simulink model "IEEE24bus_simplified"  (R2019b)
settings: Solver=ode23tb  StartTime=0.0  StopTime=100  MaxStep=1/60  RelTol=1e-4  AbsTol=1e-3  EnableMultiTasking=on
PreLoadFcn:
  | RTS96_data
values from neighbouring files (symbols this model uses):
  Efmax = 5    [IEEE24_bus.m]    (also in IEEE24bus_simplified_benchmark.m)
  Efmin = -5    [IEEE24_bus.m]    (also in IEEE24bus_simplified_benchmark.m)
  EXc_sys = [     0.06  25  0.2    0.0505  0.5685   0 0   0.091  0.35 ... (first row only)    [IEEE24bus_simplified_benchmark.m]
  FH1 = 12    [IEEE24bus_simplified_benchmark.m]
  FI1 = .9    (= 0.9)    [IEEE24bus_simplified_benchmark.m]
  FL1 = .1    (= 0.1)    [IEEE24bus_simplified_benchmark.m]
  KH1 = 100    [IEEE24bus_simplified_benchmark.m]
  KI1 = 1    [IEEE24_bus.m]    (also in IEEE24bus_simplified_benchmark.m = 20)
  KL1 = 10    [IEEE24bus_simplified_benchmark.m]
undefined symbols (not defined in the file or in its folder): D1, Delta
libraries: powerlib x157, sps_avr x11, powerlib_extras x1
(part 2 of 3)

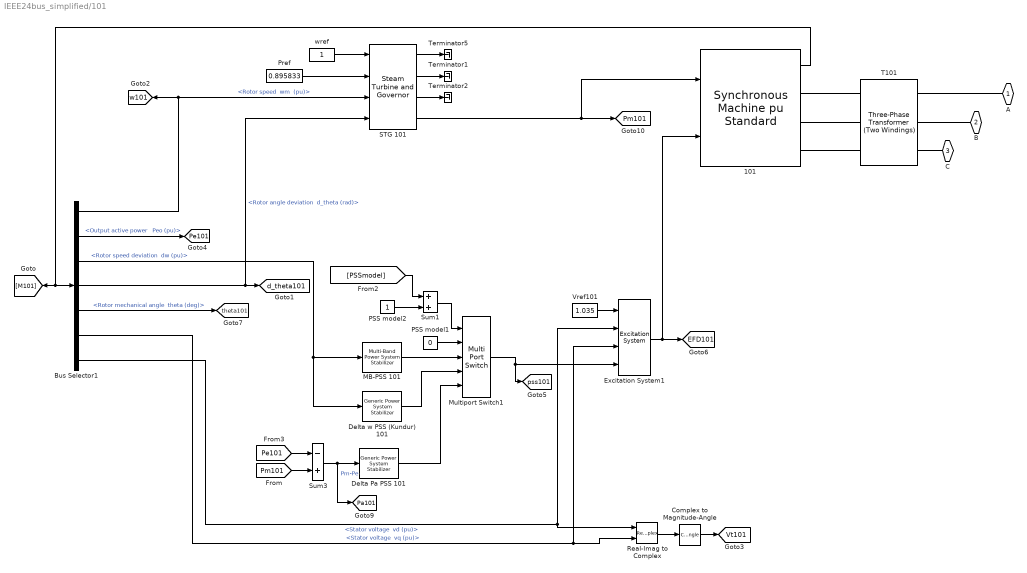
== system IEEE24bus_simplified/101 ==
  101 : powerlib/Machines/Synchronous Machine pu Standard  RequirementInfo={'other' '..\..\..\..\public\documents\just test.xlsx' '@Simulink_requirement_item_1' 'true' '' '' } %GIDa_22814801_0845_46e3_8641_b30c20268729  PresetModel=No  MechanicalLoad=Mechanical power Pm  ShowDetailedParameters=on  RotorType=Round  Units=per unit standard parameters  MeasurementBus=off  NominalParameters="[ 192E6  18000  60]"  Reactances1="[ 1.65  0.232  0.171  1.59  0.38  0.171  0.102 ]"  Reactances2="[ 1.651, 0.232, 0.171, 1.590,  0.171,  0.102 ]"  dAxisTimeConstants=Open-circuit  qAxisTimeConstants=Open-circuit  TimeConstants1="[  5.9  0.033  0.023  ]"  TimeConstants2="[ 5.9  0.033  0.735  0.078 ]"  TimeConstants3="[  5.9  0.033  0.023  ]"  TimeConstants4=[ 8.0, 0.03, 0.3371, 0.0295 ]  TimeConstants5=[ 1.01, 0.053, 0.1 ]  TimeConstants6=[ 1.3201, 0.023, 1.0, 0.07 ]  TimeConstants7="[  1.01  0.053  0.051266  ]"  TimeConstants8=[ 1.3201, 0.0231, 0.3371, 0.0295 ]  StatorResistance=0.0026  Mechanical="[ 960/233 0  4 ]"  PolePairs=4  InitialConditions=[0 -54.7243 0.868552 0.868552 0.868552 -19.5576 -139.558 100.442 1.8373]  SetSaturation=off  Saturation=[0.6404,0.7127,0.8441,0.9214,0.9956,1.082,1.19,1.316,1.457;0.7,0.7698,0.8872,0.9466,0.9969,1.046,1.1,1.151,1.201]  LoadFlowParameters=[1 172000000 18630 0 0]  TsPowergui=0  TsBlock=-1  IterativeModel=Forward Euler  IterativeDiscreteModel=Trapezoidal non iterative  BusType=PV  Pref=172E6  Qref=0  Qmin=-50E6  Qmax=80e6  PLF=0  QLF=0
      settings: SourceProductName=Simscape Electrical
  Bus Selector1 : BusSelector  OutputSignals="Mechanical.Rotor speed  wm  (pu),Output active power   Peo (pu),Mechanical.Rotor speed deviation  dw (pu),Mechanical.Rotor angle deviation  d_theta (rad),Mechanical.Rotor mechanical angle  theta (deg),dq0 components.Stator voltage  vq (pu),dq0 components.Stator voltage  vd (pu)"
  Complex to Magnitude-Angle : ComplexToMagnitudeAngle  Output=Magnitude
  Delta Pa PSS 101 : powerlib/Machines/Generic Power System Stabilizer  Tsensor=15e-3  K=2.5*1.25  Twashout=1  Tleadlag1=[60e-3 1]  Tleadlag2=[0 0]  VSlimits=[-0.15 0.15]  Vinit=0  Plot_On=off  MagdB_On=on  FreqRange=logspace(-2,2,500)
      settings: SourceProductName=Simscape Electrical  SourceProductBaseCode=PS
  Delta w PSS (Kundur) 101 : powerlib/Machines/Generic Power System Stabilizer  Tsensor=15e-3  K=30  Twashout=10  Tleadlag1=[50e-3 20e-3]  Tleadlag2=[3 5.4]  VSlimits=[-0.15 0.15]  Vinit=0  Plot_On=off  MagdB_On=on  FreqRange=logspace(-2,2,500)
      settings: SourceProductName=Simscape Electrical  SourceProductBaseCode=PS
  Excitation System1 : sps_avr/Excitation System  tr=EXc_sys(1,1)  reg="[ EXc_sys(1,2)   EXc_sys(1,3) ]"  exc="[ EXc_sys(1,4)  EXc_sys(1,5)]"  tgr="[ EXc_sys(1,6)  EXc_sys(1,7) ]"  damp="[ EXc_sys(1,8)   EXc_sys(1,9)]"  sat=[ 0, 0 ]  lim="[ Efmin Efmax   0 ]"  v0=[1.035,1.8373]
      settings: SourceProductName=Simscape Electrical  SourceProductBaseCode=PS
  "MB-PSS 101 " : powerlib/Machines/Multi-Band Power System Stabilizer  OperationMode=Simplified settings  Kg=G1  GL=[FL1 KL1]  GI=[FI1 KI1]  GH=[FH1 KH1]  GLd=[66 66 9.4]  TcLF=[1.667 2 0 0 0 0 2 2.4 0 0 0 0 1 1]  GId=[66 66 47.6]  TcIF=[1 1 0.25 0.3 0 0 1 1 0.3 0.36 0 0 0 0]  GHd=[66 66 233]  TcHF="[0.01 0.012 0 0 0 0  0.012 0.0144 0 0 0 0 1 1]"  LIM=[.075 .15 .15 .15]  Plot_On=off  MagdB_On=off  FreqRange=logspace(-2,2,500)
      settings: SourceProductName=Simscape Electrical  SourceProductBaseCode=PS
  Multiport Switch1 : MultiPortSwitch  Inputs=4  InputSameDT=on
  PSS model1 : Constant  Value=0
  PSS model2 : Constant
  Pref : Constant  Value=0.895833
  Real-Imag to Complex : RealImagToComplex
  STG 101 : powerlib/Machines/Steam Turbine and Governor  gentype=Tandem-compound (single mass)  reg1="[ 1  0.05    0 ]"  reg2="[ 0.001  0.15 ]"  reg3="[ -0.1  0.1  0  4.496 ]"  N=3600  turb1="[ 0  10   3.3   0.5   ]"  turb2="[   0   0.36    0.36   0.28   ]"  HA="[ 0.046  1.430  1.465   0.192 ]"  KA="[ 90.44  53.88  64.59   62.94  ]"  DA="[ 0.0115  0.3575  0.3663   0.0137  ]"  ini1=0.897795  ini2=[0.779316,-31.4247]
      settings: SourceProductName=Simscape Electrical  SourceProductBaseCode=PS
  Sum1 : Sum  SaturateOnIntegerOverflow=on  InputSameDT=on  OutDataTypeStr=Inherit: Same as first input
  Sum3 : Sum  Inputs=-+  SaturateOnIntegerOverflow=on  InputSameDT=on  OutDataTypeStr=Inherit: Same as first input
  T101 : powerlib/Elements/Three-Phase Transformer (Two Windings)  Winding1Connection=Yg  Winding2Connection=Delta (D1)  CoreType=Three single-phase transformers  SetSaturation=off  Hysteresis=off  DataFile='hysteresis'  SetInitialFlux=off  Measurements=None  UNITS=pu  NominalPower=[ 236E6 , 60 ]  Winding1=[ 138e3 , 0, 0.13 ]  Winding2=[ 18e3 , 1e-6, 0 ]  Rm=500  Lm=500  L0=0.5  Saturation=[ 0,0 ; 0.0024,1.2 ; 1.0,1.52 ]  InitialFluxes=[ 0.8 , -0.8 , 0.7 ]  BreakLoop=off  DiscreteSolver=Trapezoidal iterative  DataType=off  TransfoNumber=0
      settings: SourceProductName=Simscape Electrical
  Terminator1 : Terminator
  Terminator2 : Terminator
  Terminator5 : Terminator
  Vref101 : Constant  Value=1.035
  wref : Constant
  A : PMIOPort  Side=Left
  B : PMIOPort  Port=2  Side=Left
  C : PMIOPort  Port=3  Side=Left
  tag scope: EFD101=global, Pa101=global, Pe101=global, Pm101=global, Vt101=global, d_theta101=global, pss101=global, theta101=global, w101=global
  wires:
  Bus Selector1/6 -> Real-Imag to Complex/2, Excitation System1/3  "<Stator voltage  vq (pu)>"
  Bus Selector1/7 -> Real-Imag to Complex/1, Excitation System1/2  "<Stator voltage  vd (pu)>"
  wref/1 -> STG 101/1
  Vref101/1 -> Excitation System1/1
  Pref/1 -> STG 101/2
  Bus Selector1/4 -> STG 101/4, [d_theta101]  "<Rotor angle deviation  d_theta (rad)>"
  101/1 -> Bus Selector1/1, [M101]
  STG 101/1 -> Terminator5/1
  Bus Selector1/1 -> STG 101/3, [w101]  "<Rotor speed  wm  (pu)>"
  Real-Imag to Complex/1 -> Complex to Magnitude-Angle/1
  Complex to Magnitude-Angle/1 -> [Vt101]
  PSS model2/1 -> Sum1/2
  Sum1/1 -> Multiport Switch1/1
  Excitation System1/1 -> 101/2, [EFD101]
  Multiport Switch1/1 -> Excitation System1/4, [pss101]
  [PSSmodel] -> Sum1/1
  PSS model1/1 -> Multiport Switch1/2
  "MB-PSS 101 "/1 -> Multiport Switch1/3
  Bus Selector1/5 -> [theta101]  "<Rotor mechanical angle  theta (deg)>"
  Bus Selector1/2 -> [Pe101]  "<Output active power   Peo (pu)>"
  STG 101/2 -> Terminator1/1
  STG 101/3 -> Terminator2/1
  Bus Selector1/3 -> Delta w PSS (Kundur) 101/1, "MB-PSS 101 "/1  "<Rotor speed deviation  dw (pu)>"
  Sum3/1 -> [Pa101], Delta Pa PSS 101/1  "Pm-Pe"
  Delta Pa PSS 101/1 -> Multiport Switch1/5
  Delta w PSS (Kundur) 101/1 -> Multiport Switch1/4
  [Pm101] -> Sum3/2
  [Pe101] -> Sum3/1
  STG 101/4 -> 101/1, [Pm101]
  connections:
  101/RConn2 -- T101/RConn2
  101/RConn1 -- T101/RConn1
  101/RConn3 -- T101/RConn3
  C/RConn1 -- T101/LConn3
  B/RConn1 -- T101/LConn2
  A/RConn1 -- T101/LConn1

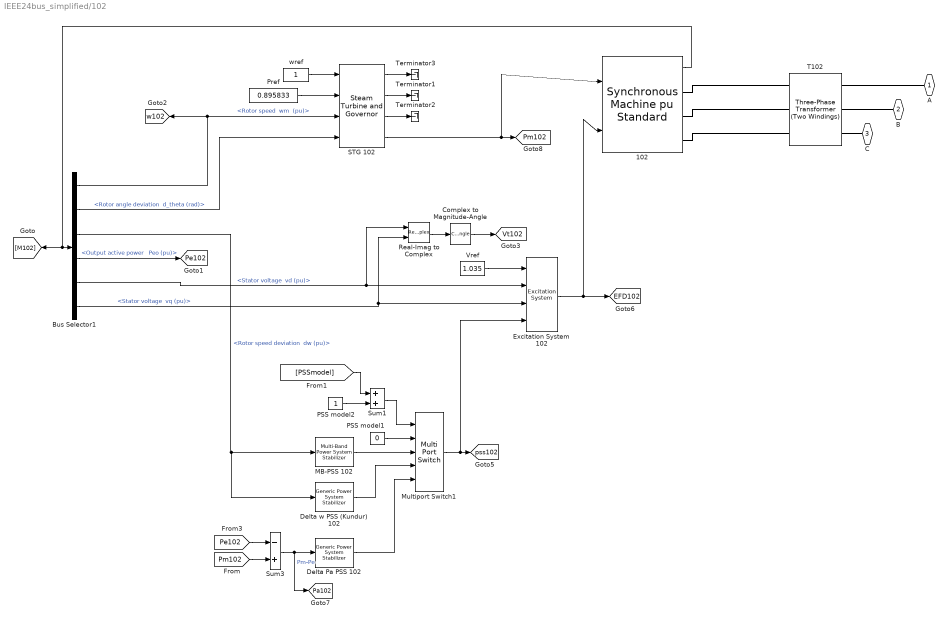
== system IEEE24bus_simplified/102 ==
  102 : powerlib/Machines/Synchronous Machine pu Standard  PresetModel=No  MechanicalLoad=Mechanical power Pm  ShowDetailedParameters=on  RotorType=Round  Units=per unit standard parameters  MeasurementBus=off  NominalParameters="[ 192E6  18000  60]"  Reactances1="[ 1.65  0.232  0.171  1.59  0.38  0.171  0.102 ]"  Reactances2="[ 1.651, 0.232, 0.171, 1.590,  0.171,  0.102 ]"  dAxisTimeConstants=Open-circuit  qAxisTimeConstants=Open-circuit  TimeConstants1="[  5.9  0.033  0.023  ]"  TimeConstants2="[ 5.9  0.033  0.735  0.078 ]"  TimeConstants3="[  5.9  0.033  0.023  ]"  TimeConstants4=[ 8.0, 0.03, 0.3371, 0.0295 ]  TimeConstants5=[ 1.01, 0.053, 0.1 ]  TimeConstants6=[ 1.3201, 0.023, 1.0, 0.07 ]  TimeConstants7="[  1.01  0.053  0.051266  ]"  TimeConstants8=[ 1.3201, 0.0231, 0.3371, 0.0295 ]  StatorResistance=0.0026  Mechanical="[ 960/233 0  4 ]"  PolePairs=4  InitialConditions=[0 -53.6767 0.866594 0.866594 0.866594 -17.7339 -137.734 102.266 1.80706]  SetSaturation=off  Saturation=[0.6404,0.7127,0.8441,0.9214,0.9956,1.082,1.19,1.316,1.457;0.7,0.7698,0.8872,0.9466,0.9969,1.046,1.1,1.151,1.201]  LoadFlowParameters=[1 172000000 18630 0 0]  TsPowergui=0  TsBlock=-1  IterativeModel=Forward Euler  IterativeDiscreteModel=Trapezoidal non iterative  BusType=PV  Pref=172E6  Qref=0  Qmin=-50e6  Qmax=80E6  PLF=0  QLF=0
      settings: SourceProductName=Simscape Electrical
  Bus Selector1 : BusSelector  OutputSignals="Mechanical.Rotor speed  wm  (pu),Mechanical.Rotor angle deviation  d_theta (rad),Mechanical.Rotor speed deviation  dw (pu),Output active power   Peo (pu),dq0 components.Stator voltage  vd (pu),dq0 components.Stator voltage  vq (pu)"
  Complex to Magnitude-Angle : ComplexToMagnitudeAngle  Output=Magnitude
  Delta Pa PSS 102 : powerlib/Machines/Generic Power System Stabilizer  Tsensor=15e-3  K=2.5*1.25  Twashout=1  Tleadlag1=[60e-3 1]  Tleadlag2=[0 0]  VSlimits=[-0.15 0.15]  Vinit=0  Plot_On=off  MagdB_On=on  FreqRange=logspace(-2,2,500)
      settings: SourceProductName=Simscape Electrical  SourceProductBaseCode=PS
  Delta w PSS (Kundur) 102 : powerlib/Machines/Generic Power System Stabilizer  Tsensor=15e-3  K=30  Twashout=10  Tleadlag1=[50e-3 20e-3]  Tleadlag2=[3 5.4]  VSlimits=[-0.15 0.15]  Vinit=0  Plot_On=off  MagdB_On=on  FreqRange=logspace(-2,2,500)
      settings: SourceProductName=Simscape Electrical  SourceProductBaseCode=PS
  Excitation System 102 : sps_avr/Excitation System  tr=EXc_sys(2,1)  reg="[ EXc_sys(2,2)   EXc_sys(2,3) ]"  exc="[ EXc_sys(2,4)  EXc_sys(2,5)]"  tgr="[ EXc_sys(2,6)  EXc_sys(2,7) ]"  damp="[ EXc_sys(2,8)   EXc_sys(2,9)]"  sat=[ 0, 0 ]  lim="[ Efmin Efmax   0 ]"  v0=[1.035,1.80706]
      settings: SourceProductName=Simscape Electrical  SourceProductBaseCode=PS
  "MB-PSS 102 " : powerlib/Machines/Multi-Band Power System Stabilizer  OperationMode=Simplified settings  Kg=G1  GL=[FL1 KL1]  GI=[FI1 KI1]  GH=[FH1 KH1]  GLd=[66 66 9.4]  TcLF=[1.667 2 0 0 0 0 2 2.4 0 0 0 0 1 1]  GId=[66 66 47.6]  TcIF=[1 1 0.25 0.3 0 0 1 1 0.3 0.36 0 0 0 0]  GHd=[66 66 233]  TcHF="[0.01 0.012 0 0 0 0  0.012 0.0144 0 0 0 0 1 1]"  LIM=[.075 .15 .15 .15]  Plot_On=off  MagdB_On=off  FreqRange=logspace(-2,2,500)
      settings: SourceProductName=Simscape Electrical  SourceProductBaseCode=PS
  Multiport Switch1 : MultiPortSwitch  Inputs=4  InputSameDT=on
  PSS model1 : Constant  Value=0
  PSS model2 : Constant
  Pref : Constant  Value=0.895833
  Real-Imag to Complex : RealImagToComplex
  STG 102 : powerlib/Machines/Steam Turbine and Governor  gentype=Tandem-compound (single mass)  reg1="[ 1  0.05    0 ]"  reg2="[ 0.001  0.15 ]"  reg3="[ -0.1  0.1  0  4.496 ]"  N=3600  turb1="[ 0  10   3.3   0.5   ]"  turb2="[   0   0.36    0.36   0.28   ]"  HA="[ 0.046  1.430  1.465   0.192 ]"  KA="[ 90.44  53.88  64.59   62.94  ]"  DA="[ 0.0115  0.3575  0.3663   0.0137  ]"  ini1=0.897786  ini2=[0.779316,-31.4247]
      settings: SourceProductName=Simscape Electrical  SourceProductBaseCode=PS
  Sum1 : Sum  SaturateOnIntegerOverflow=on  InputSameDT=on  OutDataTypeStr=Inherit: Same as first input
  Sum3 : Sum  Inputs=-+  SaturateOnIntegerOverflow=on  InputSameDT=on  OutDataTypeStr=Inherit: Same as first input
  T102 : powerlib/Elements/Three-Phase Transformer (Two Windings)  Winding1Connection=Yg  Winding2Connection=Delta (D1)  CoreType=Three single-phase transformers  SetSaturation=off  Hysteresis=off  DataFile='hysteresis'  SetInitialFlux=off  Measurements=None  UNITS=pu  NominalPower="[ 236E6  , 60 ]"  Winding1=[ 138e3 , 0, .13 ]  Winding2=[ 18e3 , 1e-6 , 0 ]  Rm=500  Lm=500  L0=0.5  Saturation=[ 0,0 ; 0.0024,1.2 ; 1.0,1.52 ]  InitialFluxes=[ 0.8 , -0.8 , 0.7 ]  BreakLoop=off  DiscreteSolver=Trapezoidal iterative  DataType=off  TransfoNumber=0
      settings: SourceProductName=Simscape Electrical
  Terminator1 : Terminator
  Terminator2 : Terminator
  Terminator3 : Terminator
  Vref : Constant  Value=1.035
  wref : Constant
  A : PMIOPort  Side=Left
  B : PMIOPort  Port=2  Side=Left
  C : PMIOPort  Port=3  Side=Left
  tag scope: EFD102=global, Pa102=global, Pe102=global, Pm102=global, Vt102=global, pss102=global, w102=global
  wires:
  STG 102/1 -> Terminator3/1
  STG 102/2 -> Terminator1/1
  STG 102/3 -> Terminator2/1
  STG 102/4 -> [Pm102], 102/1
  wref/1 -> STG 102/1
  Pref/1 -> STG 102/2
  102/1 -> [M102], Bus Selector1/1
  Bus Selector1/1 -> [w102], STG 102/3  "<Rotor speed  wm  (pu)>"
  Bus Selector1/2 -> STG 102/4  "<Rotor angle deviation  d_theta (rad)>"
  Vref/1 -> Excitation System 102/1
  Bus Selector1/5 -> Real-Imag to Complex/1, Excitation System 102/2  "<Stator voltage  vd (pu)>"
  Bus Selector1/6 -> Real-Imag to Complex/2, Excitation System 102/3  "<Stator voltage  vq (pu)>"
  PSS model2/1 -> Sum1/2
  Sum1/1 -> Multiport Switch1/1
  Multiport Switch1/1 -> Excitation System 102/4, [pss102]
  [PSSmodel] -> Sum1/1
  PSS model1/1 -> Multiport Switch1/2
  "MB-PSS 102 "/1 -> Multiport Switch1/3
  Bus Selector1/4 -> [Pe102]  "<Output active power   Peo (pu)>"
  Excitation System 102/1 -> 102/2, [EFD102]
  Real-Imag to Complex/1 -> Complex to Magnitude-Angle/1
  Complex to Magnitude-Angle/1 -> [Vt102]
  Bus Selector1/3 -> Delta w PSS (Kundur) 102/1, "MB-PSS 102 "/1  "<Rotor speed deviation  dw (pu)>"
  Sum3/1 -> [Pa102], Delta Pa PSS 102/1  "Pm-Pe"
  Delta Pa PSS 102/1 -> Multiport Switch1/5
  Delta w PSS (Kundur) 102/1 -> Multiport Switch1/4
  [Pm102] -> Sum3/2
  [Pe102] -> Sum3/1
  connections:
  102/RConn3 -- T102/RConn3
  102/RConn2 -- T102/RConn2
  102/RConn1 -- T102/RConn1
  A/RConn1 -- T102/LConn1
  C/RConn1 -- T102/LConn3
  B/RConn1 -- T102/LConn2

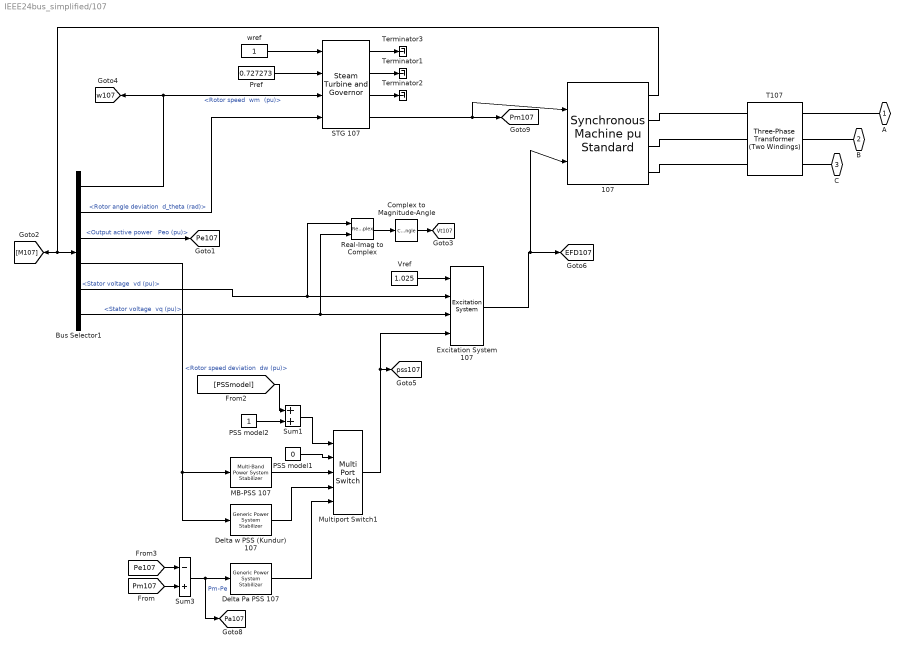
== system IEEE24bus_simplified/107 ==
  107 : powerlib/Machines/Synchronous Machine pu Standard  PresetModel=No  MechanicalLoad=Mechanical power Pm  ShowDetailedParameters=on  RotorType=Round  Units=per unit standard parameters  MeasurementBus=off  NominalParameters="[ 330E6  20000   60]"  Reactances1="[ 1.95  0.317  .2  1.92  1.12  .2  0.199 ]"  Reactances2="[ 1.9, 0.317, 0.001, 1.9,  0.001,  0.199 ]"  dAxisTimeConstants=Open-circuit  qAxisTimeConstants=Open-circuit  TimeConstants1="[  6  0.01  0.01  ]"  TimeConstants2="[ 6 .04  1.5  .08 ]"  TimeConstants3="[  6  0.01  0.01  ]"  TimeConstants4=[ 8.0, 0.03, 0.3371, 0.0295 ]  TimeConstants5=[ 1.01, 0.053, 0.1 ]  TimeConstants6=[ 1.3201, 0.023, 1.0, 0.07 ]  TimeConstants7="[  1.01  0.053  0.051266  ]"  TimeConstants8=[ 1.3201, 0.0231, 0.3371, 0.0295 ]  StatorResistance=0.0015  Mechanical="[ 992/330  0  4 ]"  PolePairs=4  InitialConditions=[0 -63.9537 0.747482 0.747482 0.747482 -34.958 -154.958 85.042 2.02909]  SetSaturation=off  Saturation=[0.6404,0.7127,0.8441,0.9214,0.9956,1.082,1.19,1.316,1.457;0.7,0.7698,0.8872,0.9466,0.9969,1.046,1.1,1.151,1.201]  LoadFlowParameters=[1 240000000 20500 0 0]  TsPowergui=0  TsBlock=-1  IterativeModel=Forward Euler  IterativeDiscreteModel=Trapezoidal non iterative  BusType=PV  Pref=240E6  Qref=0  Qmin=0  Qmax=180E6  PLF=0  QLF=0
      settings: SourceProductName=Simscape Electrical
  Bus Selector1 : BusSelector  OutputSignals="Mechanical.Rotor speed  wm  (pu),Mechanical.Rotor angle deviation  d_theta (rad),Output active power   Peo (pu),Mechanical.Rotor speed deviation  dw (pu),dq0 components.Stator voltage  vd (pu),dq0 components.Stator voltage  vq (pu)"
  Complex to Magnitude-Angle : ComplexToMagnitudeAngle  Output=Magnitude
  Delta Pa PSS 107 : powerlib/Machines/Generic Power System Stabilizer  Tsensor=15e-3  K=2.5*1.25  Twashout=1  Tleadlag1=[60e-3 1]  Tleadlag2=[0 0]  VSlimits=[-0.15 0.15]  Vinit=0  Plot_On=off  MagdB_On=on  FreqRange=logspace(-2,2,500)
      settings: SourceProductName=Simscape Electrical  SourceProductBaseCode=PS
  Delta w PSS (Kundur) 107 : powerlib/Machines/Generic Power System Stabilizer  Tsensor=15e-3  K=30  Twashout=10  Tleadlag1=[50e-3 20e-3]  Tleadlag2=[3 5.4]  VSlimits=[-0.15 0.15]  Vinit=0  Plot_On=off  MagdB_On=on  FreqRange=logspace(-2,2,500)
      settings: SourceProductName=Simscape Electrical  SourceProductBaseCode=PS
  Excitation System 107 : sps_avr/Excitation System  tr=EXc_sys(3,1)  reg="[ EXc_sys(3,2)   EXc_sys(3,3) ]"  exc="[ EXc_sys(3,4)  EXc_sys(3,5)]"  tgr="[ EXc_sys(3,6)  EXc_sys(3,7) ]"  damp="[ EXc_sys(3,8)   EXc_sys(3,9)]"  sat=[ 0, 0 ]  lim="[ Efmin Efmax   0 ]"  v0=[1.025,2.02909]
      settings: SourceProductName=Simscape Electrical  SourceProductBaseCode=PS
  MB-PSS 107 : powerlib/Machines/Multi-Band Power System Stabilizer  OperationMode=Simplified settings  Kg=G1  GL=[FL1 KL1]  GI=[FI1 KI1]  GH=[FH1 KH1]  GLd=[66 66 9.4]  TcLF=[1.667 2 0 0 0 0 2 2.4 0 0 0 0 1 1]  GId=[66 66 47.6]  TcIF=[1 1 0.25 0.3 0 0 1 1 0.3 0.36 0 0 0 0]  GHd=[66 66 233]  TcHF="[0.01 0.012 0 0 0 0  0.012 0.0144 0 0 0 0 1 1]"  LIM=[.075 .15 .15 .15]  Plot_On=off  MagdB_On=off  FreqRange=logspace(-2,2,500)
      settings: SourceProductName=Simscape Electrical  SourceProductBaseCode=PS
  Multiport Switch1 : MultiPortSwitch  Inputs=4  InputSameDT=on
  PSS model1 : Constant  Value=0
  PSS model2 : Constant
  Pref : Constant  Value=0.727273
  Real-Imag to Complex : RealImagToComplex
  STG 107 : powerlib/Machines/Steam Turbine and Governor  gentype=Tandem-compound (single mass)  reg1="[ 1  0.05    0 ]"  reg2="[ 0.001  0.15 ]"  reg3="[ -0.1  0.1  0  4.496 ]"  N=3600  turb1="[ 0  10   3.3   0.5   ]"  turb2="[   0   0.36    0.36   0.28   ]"  HA="[ 0.046  1.430  1.465   0.192 ]"  KA="[ 90.44  53.88  64.59   62.94  ]"  DA="[ 0.0115  0.3575  0.3663   0.0137  ]"  ini1=0.728111  ini2=[0.779316,-31.4247]
      settings: SourceProductName=Simscape Electrical  SourceProductBaseCode=PS
  Sum1 : Sum  SaturateOnIntegerOverflow=on  InputSameDT=on  OutDataTypeStr=Inherit: Same as first input
  Sum3 : Sum  Inputs=-+  SaturateOnIntegerOverflow=on  InputSameDT=on  OutDataTypeStr=Inherit: Same as first input
  T107 : powerlib/Elements/Three-Phase Transformer (Two Windings)  Winding1Connection=Yg  Winding2Connection=Delta (D1)  CoreType=Three single-phase transformers  SetSaturation=off  Hysteresis=off  DataFile='hysteresis'  SetInitialFlux=off  Measurements=None  UNITS=pu  NominalPower=[ 354E6 , 60 ]  Winding1="[ 138e3 , 0,  0.13 ]"  Winding2=[ 20e3 , 1e-6 , 0 ]  Rm=500  Lm=500  L0=0.5  Saturation=[ 0,0 ; 0.0024,1.2 ; 1.0,1.52 ]  InitialFluxes=[ 0.8 , -0.8 , 0.7 ]  BreakLoop=off  DiscreteSolver=Trapezoidal iterative  DataType=off  TransfoNumber=0
      settings: SourceProductName=Simscape Electrical
  Terminator1 : Terminator
  Terminator2 : Terminator
  Terminator3 : Terminator
  Vref : Constant  Value=1.025
  wref : Constant
  A : PMIOPort  Side=Left
  B : PMIOPort  Port=2  Side=Left
  C : PMIOPort  Port=3  Side=Left
  tag scope: EFD107=global, Pa107=global, Pe107=global, Pm107=global, Vt107=global, pss107=global, w107=global
  wires:
  Excitation System 107/1 -> 107/2, [EFD107]
  Vref/1 -> Excitation System 107/1
  107/1 -> [M107], Bus Selector1/1
  STG 107/1 -> Terminator3/1
  STG 107/2 -> Terminator1/1
  STG 107/3 -> Terminator2/1
  STG 107/4 -> [Pm107], 107/1
  Pref/1 -> STG 107/2
  wref/1 -> STG 107/1
  Bus Selector1/1 -> [w107], STG 107/3  "<Rotor speed  wm  (pu)>"
  Bus Selector1/2 -> STG 107/4  "<Rotor angle deviation  d_theta (rad)>"
  PSS model2/1 -> Sum1/2
  Sum1/1 -> Multiport Switch1/1
  Multiport Switch1/1 -> Excitation System 107/4, [pss107]
  [PSSmodel] -> Sum1/1
  PSS model1/1 -> Multiport Switch1/2
  MB-PSS 107/1 -> Multiport Switch1/3
  Bus Selector1/3 -> [Pe107]  "<Output active power   Peo (pu)>"
  Bus Selector1/5 -> Real-Imag to Complex/1, Excitation System 107/2  "<Stator voltage  vd (pu)>"
  Bus Selector1/6 -> Real-Imag to Complex/2, Excitation System 107/3  "<Stator voltage  vq (pu)>"
  Real-Imag to Complex/1 -> Complex to Magnitude-Angle/1
  Complex to Magnitude-Angle/1 -> [Vt107]
  Bus Selector1/4 -> Delta w PSS (Kundur) 107/1, MB-PSS 107/1  "<Rotor speed deviation  dw (pu)>"
  Sum3/1 -> [Pa107], Delta Pa PSS 107/1  "Pm-Pe"
  Delta Pa PSS 107/1 -> Multiport Switch1/5
  Delta w PSS (Kundur) 107/1 -> Multiport Switch1/4
  [Pm107] -> Sum3/2
  [Pe107] -> Sum3/1
  connections:
  107/RConn3 -- T107/RConn3
  T107/LConn2 -- B/RConn1
  107/RConn2 -- T107/RConn2
  T107/LConn1 -- A/RConn1
  107/RConn1 -- T107/RConn1
  T107/LConn3 -- C/RConn1

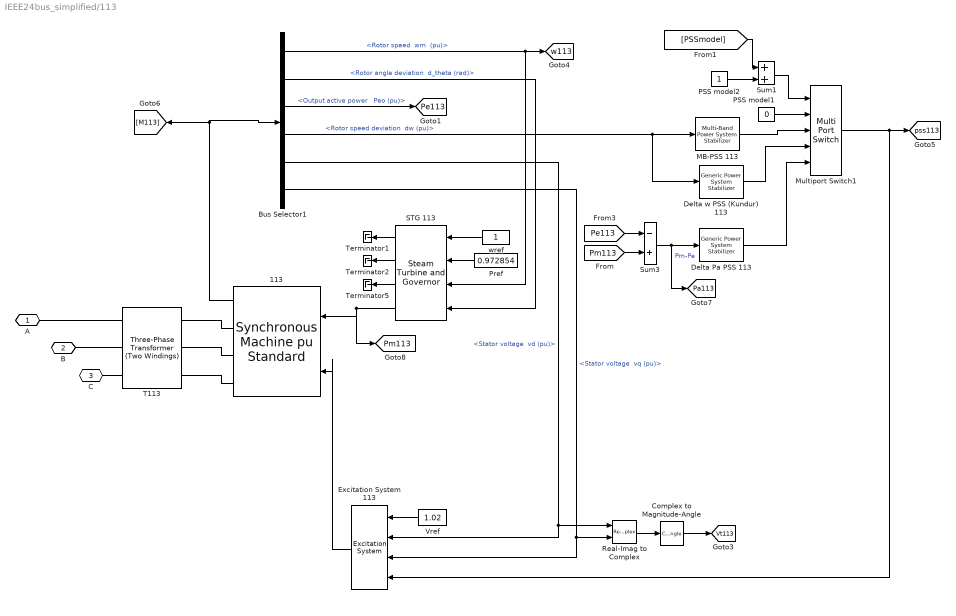
== system IEEE24bus_simplified/113 ==
  113 : powerlib/Machines/Synchronous Machine pu Standard  PresetModel=No  MechanicalLoad=Mechanical power Pm  ShowDetailedParameters=on  RotorType=Round  Units=per unit standard parameters  MeasurementBus=off  NominalParameters="[650E6  22e3   60]"  Reactances1="[ 2.11  0.28  0.215  2.02  0.49  0.215   0.155 ]"  Reactances2="[ 2.110, 0.280, 0.215, 2.020,  0.215,  0.155 ]"  dAxisTimeConstants=Open-circuit  qAxisTimeConstants=Open-circuit  TimeConstants1="[  4.2  0.032  0.0225  ]"  TimeConstants2="[ 4.2  0.032  0.565  0.062 ]"  TimeConstants3="[  4.2  0.032  0.0225  ]"  TimeConstants4=[ 8.0, 0.03, 0.3371, 0.0295 ]  TimeConstants5=[ 1.01, 0.053, 0.1 ]  TimeConstants6=[ 1.3201, 0.023, 1.0, 0.07 ]  TimeConstants7="[  1.01  0.053  0.051266  ]"  TimeConstants8=[ 1.3201, 0.0231, 0.3371, 0.0295 ]  StatorResistance=0.0046  Mechanical="[ 1368/590 0  4 ]"  PolePairs=4  InitialConditions=[0 -36.1143 0.972214 0.972214 0.972214 -11.1758 -131.176 108.824 2.46318]  SetSaturation=off  Saturation=[0.6404,0.7127,0.8441,0.9214,0.9956,1.082,1.19,1.316,1.457;0.7,0.7698,0.8872,0.9466,0.9969,1.046,1.1,1.151,1.201]  LoadFlowParameters=[2 259000000 22440 0 0]  TsPowergui=0  TsBlock=-1  IterativeModel=Forward Euler  IterativeDiscreteModel=Trapezoidal non iterative  BusType=swing  Pref=285E6  Qref=0  Qmin=0  Qmax=240E6  PLF=0  QLF=0
      settings: SourceProductName=Simscape Electrical
  Bus Selector1 : BusSelector  OutputSignals="Mechanical.Rotor speed  wm  (pu),Mechanical.Rotor angle deviation  d_theta (rad),Output active power   Peo (pu),Mechanical.Rotor speed deviation  dw (pu),dq0 components.Stator voltage  vd (pu),dq0 components.Stator voltage  vq (pu)"
  Complex to Magnitude-Angle : ComplexToMagnitudeAngle  Output=Magnitude
  Delta Pa PSS 113 : powerlib/Machines/Generic Power System Stabilizer  Tsensor=15e-3  K=2.5*1.25  Twashout=1  Tleadlag1=[60e-3 1]  Tleadlag2=[0 0]  VSlimits=[-0.15 0.15]  Vinit=0  Plot_On=off  MagdB_On=on  FreqRange=logspace(-2,2,500)
      settings: SourceProductName=Simscape Electrical  SourceProductBaseCode=PS
  Delta w PSS (Kundur) 113 : powerlib/Machines/Generic Power System Stabilizer  Tsensor=15e-3  K=30  Twashout=10  Tleadlag1=[50e-3 20e-3]  Tleadlag2=[3 5.4]  VSlimits=[-0.15 0.15]  Vinit=0  Plot_On=off  MagdB_On=on  FreqRange=logspace(-2,2,500)
      settings: SourceProductName=Simscape Electrical  SourceProductBaseCode=PS
  Excitation System 113 : sps_avr/Excitation System  tr=EXc_sys(4,1)  reg="[ EXc_sys(4,2)   EXc_sys(4,3) ]"  exc="[ EXc_sys(4,4)  EXc_sys(4,5)]"  tgr="[ EXc_sys(4,6)  EXc_sys(4,7) ]"  damp="[ EXc_sys(4,8)   EXc_sys(4,9)]"  sat=[ 0, 0 ]  lim="[ Efmin Efmax   0 ]"  v0=[1.02,2.46318]
      settings: SourceProductName=Simscape Electrical  SourceProductBaseCode=PS
  MB-PSS 113 : powerlib/Machines/Multi-Band Power System Stabilizer  OperationMode=Simplified settings  Kg=G1  GL=[FL1 KL1]  GI=[FI1 KI1]  GH=[FH1 KH1]  GLd=[66 66 9.4]  TcLF=[1.667 2 0 0 0 0 2 2.4 0 0 0 0 1 1]  GId=[66 66 47.6]  TcIF=[1 1 0.25 0.3 0 0 1 1 0.3 0.36 0 0 0 0]  GHd=[66 66 233]  TcHF="[0.01 0.012 0 0 0 0  0.012 0.0144 0 0 0 0 1 1]"  LIM=[.075 .15 .15 .15]  Plot_On=off  MagdB_On=off  FreqRange=logspace(-2,2,500)
      settings: SourceProductName=Simscape Electrical  SourceProductBaseCode=PS
  Multiport Switch1 : MultiPortSwitch  Inputs=4  InputSameDT=on
  PSS model1 : Constant  Value=0
  PSS model2 : Constant
  Pref : Constant  Value=0.972854
  Real-Imag to Complex : RealImagToComplex
  STG 113 : powerlib/Machines/Steam Turbine and Governor  gentype=Tandem-compound (single mass)  reg1="[ 1  0.05    0 ]"  reg2="[ 0.001  0.15 ]"  reg3="[ -0.1  0.1  0  4.496 ]"  N=3600  turb1="[ 0  10   3.3   0.5   ]"  turb2="[   0   0.36    0.36   0.28   ]"  HA="[ 0.046  1.430  1.465   0.192 ]"  KA="[ 90.44  53.88  64.59   62.94  ]"  DA="[ 0.0115  0.3575  0.3663   0.0137  ]"  ini1=0.977202  ini2=[0.779316,-31.4247]
      settings: SourceProductName=Simscape Electrical  SourceProductBaseCode=PS
  Sum1 : Sum  SaturateOnIntegerOverflow=on  InputSameDT=on  OutDataTypeStr=Inherit: Same as first input
  Sum3 : Sum  Inputs=-+  SaturateOnIntegerOverflow=on  InputSameDT=on  OutDataTypeStr=Inherit: Same as first input
  T113 : powerlib/Elements/Three-Phase Transformer (Two Windings)  Winding1Connection=Yg  Winding2Connection=Delta (D1)  CoreType=Three single-phase transformers  SetSaturation=off  Hysteresis=off  DataFile='hysteresis'  SetInitialFlux=off  Measurements=None  UNITS=pu  NominalPower=[ 696E6 , 60 ]  Winding1=[ 230e3 , 0, .13 ]  Winding2=[ 22e3 , 1e-6 , 0 ]  Rm=500  Lm=500  L0=0.5  Saturation=[ 0,0 ; 0.0024,1.2 ; 1.0,1.52 ]  InitialFluxes=[ 0.8 , -0.8 , 0.7 ]  BreakLoop=off  DiscreteSolver=Trapezoidal iterative  DataType=off  TransfoNumber=0
      settings: SourceProductName=Simscape Electrical
  Terminator1 : Terminator
  Terminator2 : Terminator
  Terminator5 : Terminator
  Vref : Constant  Value=1.02
  wref : Constant
  A : PMIOPort  Side=Left
  B : PMIOPort  Port=2  Side=Left
  C : PMIOPort  Port=3  Side=Left
  tag scope: Pa113=global, Pe113=global, Pm113=global, Vt113=global, pss113=global, w113=global
  wires:
  113/1 -> [M113], Bus Selector1/1
  Excitation System 113/1 -> 113/2
  Vref/1 -> Excitation System 113/1
  STG 113/4 -> [Pm113], 113/1
  STG 113/3 -> Terminator5/1
  STG 113/1 -> Terminator1/1
  STG 113/2 -> Terminator2/1
  Pref/1 -> STG 113/2
  Bus Selector1/1 -> STG 113/3, [w113]  "<Rotor speed  wm  (pu)>"
  Bus Selector1/2 -> STG 113/4  "<Rotor angle deviation  d_theta (rad)>"
  wref/1 -> STG 113/1
  Bus Selector1/3 -> [Pe113]  "<Output active power   Peo (pu)>"
  PSS model2/1 -> Sum1/2
  Sum1/1 -> Multiport Switch1/1
  Multiport Switch1/1 -> Excitation System 113/4, [pss113]
  [PSSmodel] -> Sum1/1
  PSS model1/1 -> Multiport Switch1/2
  MB-PSS 113/1 -> Multiport Switch1/3
  Bus Selector1/5 -> Excitation System 113/2, Real-Imag to Complex/1  "<Stator voltage  vd (pu)>"
  Bus Selector1/6 -> Excitation System 113/3, Real-Imag to Complex/2  "<Stator voltage  vq (pu)>"
  Real-Imag to Complex/1 -> Complex to Magnitude-Angle/1
  Complex to Magnitude-Angle/1 -> [Vt113]
  Bus Selector1/4 -> Delta w PSS (Kundur) 113/1, MB-PSS 113/1  "<Rotor speed deviation  dw (pu)>"
  Sum3/1 -> [Pa113], Delta Pa PSS 113/1  "Pm-Pe"
  Delta Pa PSS 113/1 -> Multiport Switch1/5
  Delta w PSS (Kundur) 113/1 -> Multiport Switch1/4
  [Pm113] -> Sum3/2
  [Pe113] -> Sum3/1
  connections:
  113/RConn3 -- T113/RConn3
  113/RConn2 -- T113/RConn2
  113/RConn1 -- T113/RConn1
  B/RConn1 -- T113/LConn2
  C/RConn1 -- T113/LConn3
  A/RConn1 -- T113/LConn1

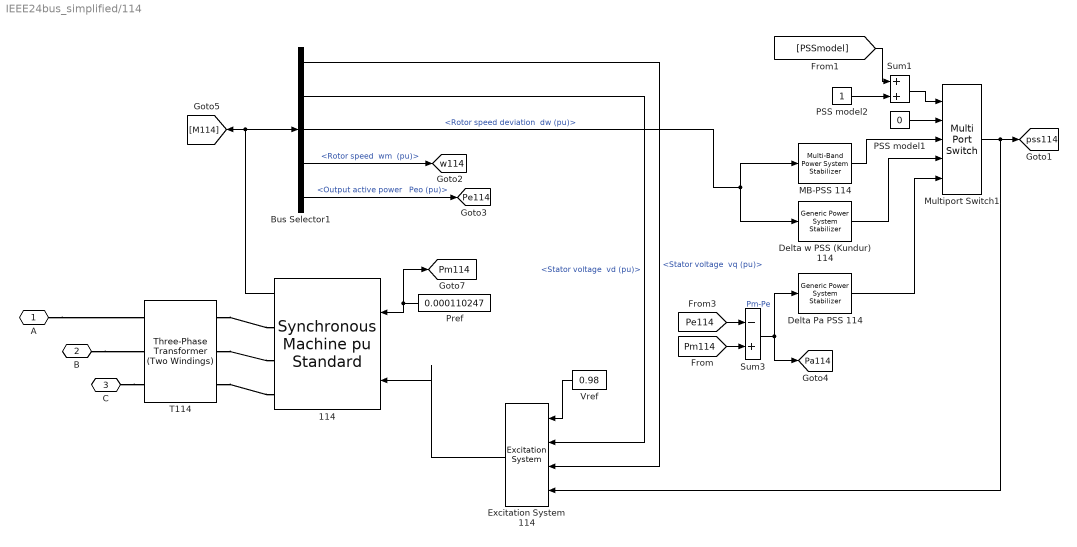
== system IEEE24bus_simplified/114 ==
  114 : powerlib/Machines/Synchronous Machine pu Standard  PresetModel=No  MechanicalLoad=Mechanical power Pm  ShowDetailedParameters=on  RotorType=Round  Units=per unit standard parameters  MeasurementBus=off  NominalParameters="[ 25E6  13.8e3   60]"  Reactances1="[ 1.769, 0.304, 0.2035, 0.855, 0.5795, 0.199,  0.1045 ]"  Reactances2="[ 1.769, 0.304, 0.2035, 0.855,  0.199,  0.1045 ]"  dAxisTimeConstants=Open-circuit  qAxisTimeConstants=Open-circuit  TimeConstants1="[  8  0.0525  0.01  ]"  TimeConstants2="[  8  0.0525  .2   0.0151  ]"  TimeConstants3="[  8  0.0525  0.001  ]"  TimeConstants4=[ 8.0, 0.03, 0.3371, 0.0295 ]  TimeConstants5=[ 1.01, 0.053, 0.1 ]  TimeConstants6=[ 1.3201, 0.023, 1.0, 0.07 ]  TimeConstants7="[  1.01  0.053  0.051266  ]"  TimeConstants8=[ 1.3201, 0.0231, 0.3371, 0.0295 ]  StatorResistance=0.0025  Mechanical="[ 30/25 0  4 ]"  PolePairs=4  InitialConditions=[0 -101.456 0.167628 0.167628 0.167628 -101.423 138.577 18.5771 1.27653]  SetSaturation=off  Saturation=[0.6404,0.7127,0.8441,0.9214,0.9956,1.082,1.19,1.316,1.457;0.7,0.7698,0.8872,0.9466,0.9969,1.046,1.1,1.151,1.201]  LoadFlowParameters=[1 1000 13524 0 0]  TsPowergui=0  TsBlock=-1  IterativeModel=Forward Euler  IterativeDiscreteModel=Trapezoidal non iterative  BusType=PV  Pref=1E3  Qref=0  Qmin=-50e6  Qmax=200E6  PLF=0  QLF=0
      settings: SourceProductName=Simscape Electrical
  Bus Selector1 : BusSelector  OutputSignals="dq0 components.Stator voltage  vq (pu),dq0 components.Stator voltage  vd (pu),Mechanical.Rotor speed deviation  dw (pu),Mechanical.Rotor speed  wm  (pu),Output active power   Peo (pu)"
  Delta Pa PSS 114 : powerlib/Machines/Generic Power System Stabilizer  Tsensor=15e-3  K=2.5*1.25  Twashout=1  Tleadlag1=[60e-3 1]  Tleadlag2=[0 0]  VSlimits=[-0.15 0.15]  Vinit=0  Plot_On=off  MagdB_On=on  FreqRange=logspace(-2,2,500)
      settings: SourceProductName=Simscape Electrical  SourceProductBaseCode=PS
  Delta w PSS (Kundur) 114 : powerlib/Machines/Generic Power System Stabilizer  Tsensor=15e-3  K=30  Twashout=10  Tleadlag1=[50e-3 20e-3]  Tleadlag2=[3 5.4]  VSlimits=[-0.15 0.15]  Vinit=0  Plot_On=off  MagdB_On=on  FreqRange=logspace(-2,2,500)
      settings: SourceProductName=Simscape Electrical  SourceProductBaseCode=PS
  Excitation System 114 : sps_avr/Excitation System  tr=EXc_sys(5,1)  reg="[ EXc_sys(5,2)   EXc_sys(5,3) ]"  exc="[ EXc_sys(5,4)  EXc_sys(5,5)]"  tgr="[ EXc_sys(5,6)  EXc_sys(5,7) ]"  damp="[ EXc_sys(5,8)   EXc_sys(5,9)]"  sat=[ 0, 0 ]  lim="[ Efmin Efmax   0 ]"  v0=[0.98,1.27653]
      settings: SourceProductName=Simscape Electrical  SourceProductBaseCode=PS
  "MB-PSS 114 " : powerlib/Machines/Multi-Band Power System Stabilizer  OperationMode=Simplified settings  Kg=G1  GL=[FL1 KL1]  GI=[FI1 KI1]  GH=[FH1 KH1]  GLd=[66 66 9.4]  TcLF=[1.667 2 0 0 0 0 2 2.4 0 0 0 0 1 1]  GId=[66 66 47.6]  TcIF=[1 1 0.25 0.3 0 0 1 1 0.3 0.36 0 0 0 0]  GHd=[66 66 233]  TcHF="[0.01 0.012 0 0 0 0  0.012 0.0144 0 0 0 0 1 1]"  LIM=[.075 .15 .15 .15]  Plot_On=off  MagdB_On=off  FreqRange=logspace(-2,2,500)
      settings: SourceProductName=Simscape Electrical  SourceProductBaseCode=PS
  Multiport Switch1 : MultiPortSwitch  Inputs=4  InputSameDT=on
  PSS model1 : Constant  Value=0
  PSS model2 : Constant
  Pref : Constant  Value=0.000110247
  Sum1 : Sum  SaturateOnIntegerOverflow=on  InputSameDT=on  OutDataTypeStr=Inherit: Same as first input
  Sum3 : Sum  Inputs=-+  SaturateOnIntegerOverflow=on  InputSameDT=on  OutDataTypeStr=Inherit: Same as first input
  T114 : powerlib/Elements/Three-Phase Transformer (Two Windings)  Winding1Connection=Yg  Winding2Connection=Delta (D1)  CoreType=Three single-phase transformers  SetSaturation=off  Hysteresis=off  DataFile='hysteresis'  SetInitialFlux=off  Measurements=None  UNITS=pu  NominalPower=[ 250e6 , 60 ]  Winding1=[ 230e3 , 0, .13 ]  Winding2=[ 13.8e3 , 1e-6 , 0 ]  Rm=500  Lm=500  L0=0.5  Saturation=[ 0,0 ; 0.0024,1.2 ; 1.0,1.52 ]  InitialFluxes=[ 0.8 , -0.8 , 0.7 ]  BreakLoop=off  DiscreteSolver=Trapezoidal iterative  DataType=off  TransfoNumber=0
      settings: SourceProductName=Simscape Electrical
  Vref : Constant  Value=0.98
  A : PMIOPort  Side=Left
  B : PMIOPort  Port=2  Side=Left
  C : PMIOPort  Port=3  Side=Left
  tag scope: Pa114=global, Pe114=global, Pm114=global, pss114=global, w114=global
  wires:
  114/1 -> [M114], Bus Selector1/1
  Bus Selector1/1 -> Excitation System 114/3  "<Stator voltage  vq (pu)>"
  Bus Selector1/2 -> Excitation System 114/2  "<Stator voltage  vd (pu)>"
  Vref/1 -> Excitation System 114/1
  Excitation System 114/1 -> 114/2
  Pref/1 -> [Pm114], 114/1
  PSS model2/1 -> Sum1/2
  Sum1/1 -> Multiport Switch1/1
  Multiport Switch1/1 -> Excitation System 114/4, [pss114]
  [PSSmodel] -> Sum1/1
  PSS model1/1 -> Multiport Switch1/2
  "MB-PSS 114 "/1 -> Multiport Switch1/3
  Bus Selector1/4 -> [w114]  "<Rotor speed  wm  (pu)>"
  Bus Selector1/3 -> Delta w PSS (Kundur) 114/1, "MB-PSS 114 "/1  "<Rotor speed deviation  dw (pu)>"
  Sum3/1 -> Delta Pa PSS 114/1, [Pa114]  "Pm-Pe"
  Delta Pa PSS 114/1 -> Multiport Switch1/5
  Delta w PSS (Kundur) 114/1 -> Multiport Switch1/4
  [Pm114] -> Sum3/2
  [Pe114] -> Sum3/1
  Bus Selector1/5 -> [Pe114]  "<Output active power   Peo (pu)>"
  connections:
  T114/RConn3 -- 114/RConn3
  B/RConn1 -- T114/LConn2
  T114/RConn2 -- 114/RConn2
  C/RConn1 -- T114/LConn3
  T114/RConn1 -- 114/RConn1
  A/RConn1 -- T114/LConn1

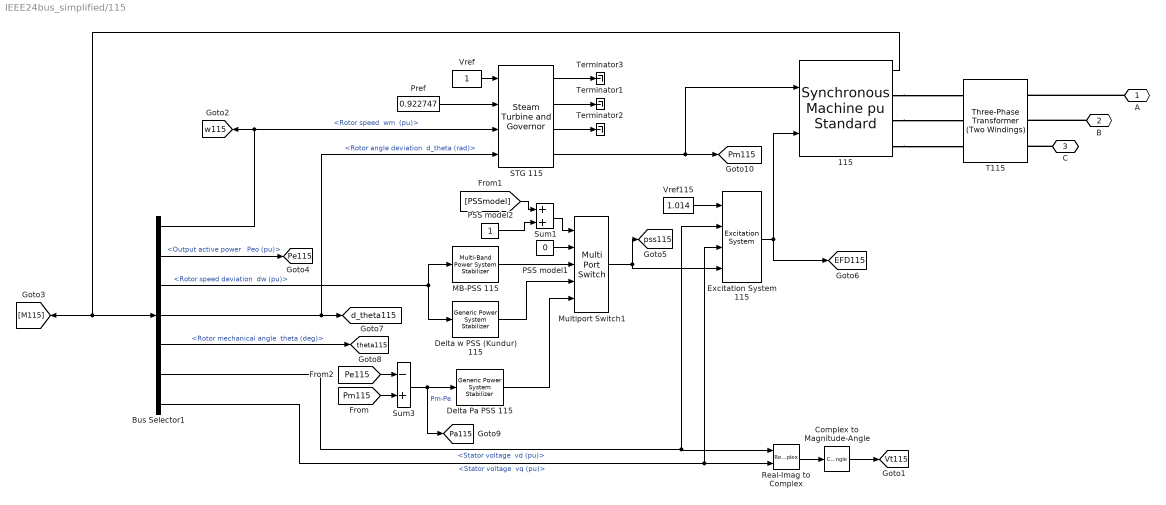
== system IEEE24bus_simplified/115 ==
  115 : powerlib/Machines/Synchronous Machine pu Standard  PresetModel=No  MechanicalLoad=Mechanical power Pm  ShowDetailedParameters=on  RotorType=Round  Units=per unit standard parameters  MeasurementBus=off  NominalParameters="[ 233e6  20e3   60]"  Reactances1="[ 1.569, 0.324, 0.249, 1.548,  0.918, 0.248,  0.204 ]"  Reactances2="[ 1.569, 0.324, 0.249, 1.548,  0.248,  0.204 ]"  dAxisTimeConstants=Open-circuit  qAxisTimeConstants=Open-circuit  TimeConstants1="[  5.140  0.0437  0.01  ]"  TimeConstants2="[  5.140  0.0437  1.5  .141 ]"  TimeConstants3="[  5.140  0.0437  0.01  ]"  TimeConstants4=[ 8.0, 0.03, 0.3371, 0.0295 ]  TimeConstants5=[ 1.01, 0.053, 0.1 ]  TimeConstants6=[ 1.3201, 0.023, 1.0, 0.07 ]  TimeConstants7="[  1.01  0.053  0.051266  ]"  TimeConstants8=[ 1.3201, 0.0231, 0.3371, 0.0295 ]  StatorResistance=0.0016  Mechanical="[ 960.5/(233) 0  4 ]"  PolePairs=4  InitialConditions=[0 -39.2481 0.931148 0.931148 0.931148 -8.31725 -128.317 111.683 1.94763]  SetSaturation=off  Saturation=[0.6404,0.7127,0.8441,0.9214,0.9956,1.082,1.19,1.316,1.457;0.7,0.7698,0.8872,0.9466,0.9969,1.046,1.1,1.151,1.201]  LoadFlowParameters=[1 215000000 20280 0 0]  TsPowergui=0  TsBlock=-1  IterativeModel=Forward Euler  IterativeDiscreteModel=Trapezoidal non iterative  BusType=PV  Pref=215E6  Qref=0  Qmin=-50e6  Qmax=110E6  PLF=0  QLF=0
      settings: SourceProductName=Simscape Electrical
  Bus Selector1 : BusSelector  OutputSignals="Mechanical.Rotor speed  wm  (pu),Output active power   Peo (pu),Mechanical.Rotor speed deviation  dw (pu),Mechanical.Rotor angle deviation  d_theta (rad),Mechanical.Rotor mechanical angle  theta (deg),dq0 components.Stator voltage  vd (pu),dq0 components.Stator voltage  vq (pu)"
  Complex to Magnitude-Angle : ComplexToMagnitudeAngle  Output=Magnitude
  Delta Pa PSS 115 : powerlib/Machines/Generic Power System Stabilizer  Tsensor=15e-3  K=2.5*1.25  Twashout=1  Tleadlag1=[60e-3 1]  Tleadlag2=[0 0]  VSlimits=[-0.15 0.15]  Vinit=0  Plot_On=off  MagdB_On=on  FreqRange=logspace(-2,2,500)
      settings: SourceProductName=Simscape Electrical  SourceProductBaseCode=PS
  Delta w PSS (Kundur) 115 : powerlib/Machines/Generic Power System Stabilizer  Tsensor=15e-3  K=30  Twashout=10  Tleadlag1=[50e-3 20e-3]  Tleadlag2=[3 5.4]  VSlimits=[-0.15 0.15]  Vinit=0  Plot_On=off  MagdB_On=on  FreqRange=logspace(-2,2,500)
      settings: SourceProductName=Simscape Electrical  SourceProductBaseCode=PS
  Excitation System 115 : sps_avr/Excitation System  tr=EXc_sys(6,1)  reg="[ EXc_sys(6,2)   EXc_sys(6,3) ]"  exc="[ EXc_sys(6,4)  EXc_sys(6,5)]"  tgr="[ EXc_sys(6,6)  EXc_sys(6,7) ]"  damp="[ EXc_sys(6,8)   EXc_sys(6,9)]"  sat=[ 0, 0 ]  lim="[ Efmin Efmax   0 ]"  v0=[1.014,1.94763]
      settings: SourceProductName=Simscape Electrical  SourceProductBaseCode=PS
  "MB-PSS 115 " : powerlib/Machines/Multi-Band Power System Stabilizer  OperationMode=Simplified settings  Kg=G1  GL=[FL1 KL1]  GI=[FI1 KI1]  GH=[FH1 KH1]  GLd=[66 66 9.4]  TcLF=[1.667 2 0 0 0 0 2 2.4 0 0 0 0 1 1]  GId=[66 66 47.6]  TcIF=[1 1 0.25 0.3 0 0 1 1 0.3 0.36 0 0 0 0]  GHd=[66 66 233]  TcHF="[0.01 0.012 0 0 0 0  0.012 0.0144 0 0 0 0 1 1]"  LIM=[.075 .15 .15 .15]  Plot_On=off  MagdB_On=off  FreqRange=logspace(-2,2,500)
      settings: SourceProductName=Simscape Electrical  SourceProductBaseCode=PS
  Multiport Switch1 : MultiPortSwitch  Inputs=4  InputSameDT=on
  PSS model1 : Constant  Value=0
  PSS model2 : Constant
  Pref : Constant  Value=0.922747
  Real-Imag to Complex : RealImagToComplex
  STG 115 : powerlib/Machines/Steam Turbine and Governor  gentype=Tandem-compound (single mass)  reg1="[ 1  0.05    0 ]"  reg2="[ 0.001  0.15 ]"  reg3="[ -0.1  0.1  0  4.496 ]"  N=3600  turb1="[ 0  10   3.3   0.5   ]"  turb2="[   0   0.36    0.36   0.28   ]"  HA="[ 0.046  1.430  1.465   0.192 ]"  KA="[ 90.44  53.88  64.59   62.94  ]"  DA="[ 0.0115  0.3575  0.3663   0.0137  ]"  ini1=0.924134  ini2=[0.779316,-31.4247]
      settings: SourceProductName=Simscape Electrical  SourceProductBaseCode=PS
  Sum1 : Sum  SaturateOnIntegerOverflow=on  InputSameDT=on  OutDataTypeStr=Inherit: Same as first input
  Sum3 : Sum  Inputs=-+  SaturateOnIntegerOverflow=on  InputSameDT=on  OutDataTypeStr=Inherit: Same as first input
  T115 : powerlib/Elements/Three-Phase Transformer (Two Windings)  Winding1Connection=Delta (D1)  Winding2Connection=Yg  CoreType=Three single-phase transformers  SetSaturation=off  Hysteresis=off  DataFile='hysteresis'  SetInitialFlux=off  Measurements=None  UNITS=pu  NominalPower=[ 252e6 , 60 ]  Winding1=[ 20e3 , 1e-6, 0 ]  Winding2=[ 230e3 , 0, 0.13 ]  Rm=500  Lm=500  L0=0.5  Saturation=[ 0,0 ; 0.0024,1.2 ; 1.0,1.52 ]  InitialFluxes=[ 0.8 , -0.8 , 0.7 ]  BreakLoop=off  DiscreteSolver=Trapezoidal iterative  DataType=off  TransfoNumber=0
      settings: SourceProductName=Simscape Electrical
  Terminator1 : Terminator
  Terminator2 : Terminator
  Terminator3 : Terminator
  Vref : Constant
  Vref115 : Constant  Value=1.014
  A : PMIOPort  Side=Right
  B : PMIOPort  Port=2  Side=Right
  C : PMIOPort  Port=3  Side=Right
  tag scope: EFD115=global, Pa115=global, Pe115=global, Pm115=global, Vt115=global, d_theta115=global, pss115=global, theta115=global, w115=global
  wires:
  Vref/1 -> STG 115/1
  Pref/1 -> STG 115/2
  Excitation System 115/1 -> 115/2, [EFD115]
  Bus Selector1/1 -> STG 115/3, [w115]  "<Rotor speed  wm  (pu)>"
  Bus Selector1/2 -> [Pe115]  "<Output active power   Peo (pu)>"
  Multiport Switch1/1 -> Excitation System 115/4, [pss115]
  PSS model2/1 -> Sum1/2
  Sum1/1 -> Multiport Switch1/1
  [PSSmodel] -> Sum1/1
  PSS model1/1 -> Multiport Switch1/2
  "MB-PSS 115 "/1 -> Multiport Switch1/3
  Real-Imag to Complex/1 -> Complex to Magnitude-Angle/1
  Complex to Magnitude-Angle/1 -> [Vt115]
  115/1 -> Bus Selector1/1, [M115]
  Bus Selector1/4 -> [d_theta115], STG 115/4  "<Rotor angle deviation  d_theta (rad)>"
  Bus Selector1/5 -> [theta115]  "<Rotor mechanical angle  theta (deg)>"
  Bus Selector1/6 -> Excitation System 115/2, Real-Imag to Complex/1  "<Stator voltage  vd (pu)>"
  Bus Selector1/7 -> Excitation System 115/3, Real-Imag to Complex/2  "<Stator voltage  vq (pu)>"
  STG 115/1 -> Terminator3/1
  STG 115/2 -> Terminator1/1
  STG 115/3 -> Terminator2/1
  STG 115/4 -> 115/1, [Pm115]
  Vref115/1 -> Excitation System 115/1
  Bus Selector1/3 -> Delta w PSS (Kundur) 115/1, "MB-PSS 115 "/1  "<Rotor speed deviation  dw (pu)>"
  Sum3/1 -> [Pa115], Delta Pa PSS 115/1  "Pm-Pe"
  Delta Pa PSS 115/1 -> Multiport Switch1/5
  Delta w PSS (Kundur) 115/1 -> Multiport Switch1/4
  [Pm115] -> Sum3/2
  [Pe115] -> Sum3/1
  connections:
  115/RConn3 -- T115/LConn3
  115/RConn1 -- T115/LConn1
  B/RConn1 -- T115/RConn2
  A/RConn1 -- T115/RConn1
  C/RConn1 -- T115/RConn3
  115/RConn2 -- T115/LConn2

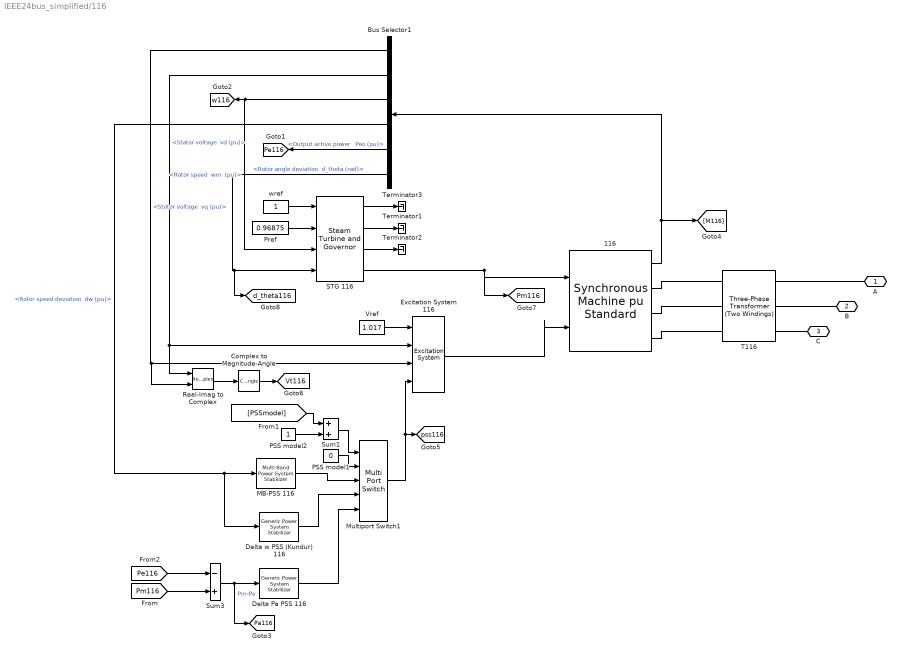
== system IEEE24bus_simplified/116 ==
  116 : powerlib/Machines/Synchronous Machine pu Standard  PresetModel=No  MechanicalLoad=Mechanical power Pm  ShowDetailedParameters=on  RotorType=Round  Units=per unit standard parameters  MeasurementBus=off  NominalParameters="[ 160E6  15e3  60]"  Reactances1="[ 1.7, 0.245, 0.185, 1.640, 0.38  0.185,  0.110 ]"  Reactances2="[ 1.7, 0.245, 0.185, 1.640,  0.185,  0.110 ]"  dAxisTimeConstants=Open-circuit  qAxisTimeConstants=Open-circuit  TimeConstants1="[  5.9  0.033  0.01  ]"  TimeConstants2=[ 5.9, 0.033, 0.74, 0.076 ]  TimeConstants3="[  5.9  0.033  0.01  ]"  TimeConstants4=[ 8.0, 0.03, 0.3371, 0.0295 ]  TimeConstants5=[ 1.01, 0.053, 0.1 ]  TimeConstants6=[ 1.3201, 0.023, 1.0, 0.07 ]  TimeConstants7="[  1.01  0.053  0.051266  ]"  TimeConstants8=[ 1.3201, 0.0231, 0.3371, 0.0295 ]  StatorResistance=0.0031  Mechanical="[ 634/(160) 0  4 ]"  PolePairs=4  InitialConditions=[0 -37.549 0.975868 0.975868 0.975868 -8.88406 -128.884 111.116 2.12717]  SetSaturation=off  Saturation=[0.6404,0.7127,0.8441,0.9214,0.9956,1.082,1.19,1.316,1.457;0.7,0.7698,0.8872,0.9466,0.9969,1.046,1.1,1.151,1.201]  LoadFlowParameters=[1 155000000 15255 0 0]  TsPowergui=0  TsBlock=-1  IterativeModel=Forward Euler  IterativeDiscreteModel=Trapezoidal non iterative  BusType=PV  Pref=155E6  Qref=0  Qmin=-50e6  Qmax=80E6  PLF=0  QLF=0
      settings: SourceProductName=Simscape Electrical
  Bus Selector1 : BusSelector  OutputSignals="dq0 components.Stator voltage  vq (pu),dq0 components.Stator voltage  vd (pu),Mechanical.Rotor speed  wm  (pu),Mechanical.Rotor speed deviation  dw (pu),Output active power   Peo (pu),Mechanical.Rotor angle deviation  d_theta (rad)"
  Complex to Magnitude-Angle : ComplexToMagnitudeAngle  Output=Magnitude
  Delta Pa PSS 116 : powerlib/Machines/Generic Power System Stabilizer  Tsensor=15e-3  K=2.5*1.25  Twashout=1  Tleadlag1=[60e-3 1]  Tleadlag2=[0 0]  VSlimits=[-0.15 0.15]  Vinit=0  Plot_On=off  MagdB_On=on  FreqRange=logspace(-2,2,500)
      settings: SourceProductName=Simscape Electrical  SourceProductBaseCode=PS
  Delta w PSS (Kundur) 116 : powerlib/Machines/Generic Power System Stabilizer  Tsensor=15e-3  K=30  Twashout=10  Tleadlag1=[50e-3 20e-3]  Tleadlag2=[3 5.4]  VSlimits=[-0.15 0.15]  Vinit=0  Plot_On=off  MagdB_On=on  FreqRange=logspace(-2,2,500)
      settings: SourceProductName=Simscape Electrical  SourceProductBaseCode=PS
  Excitation System 116 : sps_avr/Excitation System  tr=EXc_sys(7,1)  reg="[ EXc_sys(7,2)   EXc_sys(7,3) ]"  exc="[ EXc_sys(7,4)  EXc_sys(7,5)]"  tgr="[ EXc_sys(7,6)  EXc_sys(7,7) ]"  damp="[ EXc_sys(7,8)   EXc_sys(7,9)]"  sat=[ 0, 0 ]  lim="[ Efmin Efmax   0 ]"  v0=[1.017,2.12717]
      settings: SourceProductName=Simscape Electrical  SourceProductBaseCode=PS
  MB-PSS 116 : powerlib/Machines/Multi-Band Power System Stabilizer  OperationMode=Simplified settings  Kg=G1  GL=[FL1 KL1]  GI=[FI1 KI1]  GH=[FH1 KH1]  GLd=[66 66 9.4]  TcLF=[1.667 2 0 0 0 0 2 2.4 0 0 0 0 1 1]  GId=[66 66 47.6]  TcIF=[1 1 0.25 0.3 0 0 1 1 0.3 0.36 0 0 0 0]  GHd=[66 66 233]  TcHF="[0.01 0.012 0 0 0 0  0.012 0.0144 0 0 0 0 1 1]"  LIM=[.075 .15 .15 .15]  Plot_On=off  MagdB_On=off  FreqRange=logspace(-2,2,500)
      settings: SourceProductName=Simscape Electrical  SourceProductBaseCode=PS
  Multiport Switch1 : MultiPortSwitch  Inputs=4  InputSameDT=on
  PSS model1 : Constant  Value=0
  PSS model2 : Constant
  Pref : Constant  Value=0.96875
  Real-Imag to Complex : RealImagToComplex
  STG 116 : powerlib/Machines/Steam Turbine and Governor  gentype=Tandem-compound (single mass)  reg1="[ 1  0.05    0 ]"  reg2="[ 0.001  0.15 ]"  reg3="[ -0.1  0.1  0  4.496 ]"  N=3600  turb1="[ 0  10   3.3   0.5   ]"  turb2="[   0   0.36    0.36   0.28   ]"  HA="[ 0.046  1.430  1.465   0.192 ]"  KA="[ 90.44  53.88  64.59   62.94  ]"  DA="[ 0.0115  0.3575  0.3663   0.0137  ]"  ini1=0.971702  ini2=[0.779316,-31.4247]
      settings: SourceProductName=Simscape Electrical  SourceProductBaseCode=PS
  Sum1 : Sum  SaturateOnIntegerOverflow=on  InputSameDT=on  OutDataTypeStr=Inherit: Same as first input
  Sum3 : Sum  Inputs=-+  SaturateOnIntegerOverflow=on  InputSameDT=on  OutDataTypeStr=Inherit: Same as first input
  T116 : powerlib/Elements/Three-Phase Transformer (Two Windings)  Winding1Connection=Delta (D1)  Winding2Connection=Yg  CoreType=Three single-phase transformers  SetSaturation=off  Hysteresis=off  DataFile='hysteresis'  SetInitialFlux=off  Measurements=None  UNITS=pu  NominalPower=[ 182E6 , 60 ]  Winding1=[ 15e3 , 1e-6 , 0 ]  Winding2="[ 230e3 , 0,  0.13 ]"  Rm=500  Lm=500  L0=0.5  Saturation=[ 0,0 ; 0.0024,1.2 ; 1.0,1.52 ]  InitialFluxes=[ 0.8 , -0.8 , 0.7 ]  BreakLoop=off  DiscreteSolver=Trapezoidal iterative  DataType=off  TransfoNumber=0
      settings: SourceProductName=Simscape Electrical
  Terminator1 : Terminator
  Terminator2 : Terminator
  Terminator3 : Terminator
  Vref : Constant  Value=1.017
  wref : Constant
  A : PMIOPort  Side=Right
  B : PMIOPort  Port=2  Side=Right
  C : PMIOPort  Port=3  Side=Right
  tag scope: Pa116=global, Pe116=global, Pm116=global, Vt116=global, d_theta116=global, pss116=global, w116=global
  wires:
  116/1 -> Bus Selector1/1, [M116]
  Bus Selector1/1 -> Real-Imag to Complex/2, Excitation System 116/3  "<Stator voltage  vq (pu)>"
  Bus Selector1/2 -> Real-Imag to Complex/1, Excitation System 116/2  "<Stator voltage  vd (pu)>"
  wref/1 -> STG 116/1
  Pref/1 -> STG 116/2
  Excitation System 116/1 -> 116/2
  Vref/1 -> Excitation System 116/1
  Bus Selector1/3 -> STG 116/3, [w116]  "<Rotor speed  wm  (pu)>"
  PSS model2/1 -> Sum1/2
  Sum1/1 -> Multiport Switch1/1
  Multiport Switch1/1 -> Excitation System 116/4, [pss116]
  [PSSmodel] -> Sum1/1
  PSS model1/1 -> Multiport Switch1/2
  MB-PSS 116/1 -> Multiport Switch1/3
  STG 116/4 -> [Pm116], 116/1
  Bus Selector1/6 -> [d_theta116], STG 116/4  "<Rotor angle deviation  d_theta (rad)>"
  Bus Selector1/5 -> [Pe116]  "<Output active power   Peo (pu)>"
  STG 116/1 -> Terminator3/1
  STG 116/2 -> Terminator1/1
  STG 116/3 -> Terminator2/1
  Bus Selector1/4 -> Delta w PSS (Kundur) 116/1, MB-PSS 116/1  "<Rotor speed deviation  dw (pu)>"
  Sum3/1 -> [Pa116], Delta Pa PSS 116/1  "Pm-Pe"
  Delta Pa PSS 116/1 -> Multiport Switch1/5
  Delta w PSS (Kundur) 116/1 -> Multiport Switch1/4
  [Pm116] -> Sum3/2
  [Pe116] -> Sum3/1
  Real-Imag to Complex/1 -> Complex to Magnitude-Angle/1
  Complex to Magnitude-Angle/1 -> [Vt116]
  connections:
  116/RConn3 -- T116/LConn3
  116/RConn2 -- T116/LConn2
  C/RConn1 -- T116/RConn3
  B/RConn1 -- T116/RConn2
  116/RConn1 -- T116/LConn1
  A/RConn1 -- T116/RConn1
